simulink model "sim05"  (R2012b)
settings: Solver=ode45  StartTime=0.0  StopTime=40.0  RelTol=1e-3
settings Model: Creator=Administrator  LastModifiedBy=Administrator

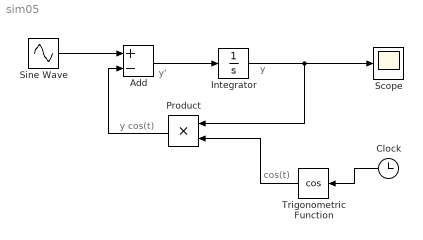
== system sim05 ==
  note: cos(t)
  note: y cos(t)
  note: y
  note: y'
  Add : Sum  Inputs=+-
  Clock : Clock
  Integrator : Integrator  InitialCondition=1
  Product : Product  RndMeth=Zero
  Scope : Scope
  Sine Wave : Sin  SampleTime=0
  Trigonometric Function : Trigonometry  Operator=cos
  wires:
  Add/1 -> Integrator/1
  Integrator/1 -> Product/1, Scope/1
  Sine Wave/1 -> Add/1
  Product/1 -> Add/2
  Trigonometric Function/1 -> Product/2
  Clock/1 -> Trigonometric Function/1
